simulink model "VDSE_2019b1"  (R2022b)
settings: Solver=ode5  StartTime=0.0  StopTime=T_simulation  FixedStep=simulation_step_time  RelTol=1e-3
values from neighbouring files (symbols this model uses):
  A = 2    [vehicle_parameters_script.m]
  bump_height = 0    [vehicle_parameters_script.m]
  bump_length = 0    [vehicle_parameters_script.m]
  bump_time = 0    [vehicle_parameters_script.m]
  cd = 0.35    [vehicle_parameters_script.m]
  cF = 5000    [vehicle_parameters_script.m]
  clF = -0.15    [vehicle_parameters_script.m]
  clR = -0.20    (= -0.2)    [vehicle_parameters_script.m]
  cp_FA = 30    [vehicle_parameters_script.m]
  cp_RA = 13    [vehicle_parameters_script.m]
  cR = 5000    [vehicle_parameters_script.m]
  ctF = tireF.VERTICAL_DAMPING    [vehicle_parameters_script.m]
  ctR = tireR.VERTICAL_DAMPING    [vehicle_parameters_script.m]
  enableDriverControl = 1    [vehicle_parameters_script.m]
  enableLongDynamics = 1    [vehicle_parameters_script.m]
  enablePowertrain = 1    [vehicle_parameters_script.m]
  g = 9.806    [vehicle_parameters_script.m]
  Gear_numbers = [1 2 3 4 5 6]    [vehicle_parameters_script.m]
  GR = [2.9 1.8 1.3 1 0.85 0.75]    [vehicle_parameters_script.m]
  hcog = 0.441    [vehicle_parameters_script.m]
  hpc = 0.0    (= 0)    [vehicle_parameters_script.m]
  hrcF = 0.3    [vehicle_parameters_script.m]
  hrcg = (hrcF*lR+hrcR*lF)/(lF+lR)    (= 0.25108)    [vehicle_parameters_script.m]
  hrcR = 0.2    [vehicle_parameters_script.m]
  huFcog = 0.32    [vehicle_parameters_script.m]
  huRcog = 0.32    [vehicle_parameters_script.m]
  i1 = 11.42    [vehicle_parameters_script.m]
  i2 = 3.727    [vehicle_parameters_script.m]
  initial_gear = 1    [vehicle_parameters_script.m]
  JwF = 2.45    [vehicle_parameters_script.m]
  JwR = 2.45    [vehicle_parameters_script.m]
  Jx = 4.12    [vehicle_parameters_script.m]
  Jy = 109.16    [vehicle_parameters_script.m]
  Jz = 105.13    [vehicle_parameters_script.m]
  kF = 40000    [vehicle_parameters_script.m]
  kR = 35000    [vehicle_parameters_script.m]
  kRF = 0    [vehicle_parameters_script.m]
  kRR = 0    [vehicle_parameters_script.m]
  ktF = tireF.VERTICAL_STIFFNESS    [vehicle_parameters_script.m]
  ktR = tireR.VERTICAL_STIFFNESS    [vehicle_parameters_script.m]
  lF = 1.223    [vehicle_parameters_script.m]
  lR = l-lF    (= 1.277)    [vehicle_parameters_script.m]
  m = 340    [vehicle_parameters_script.m]
  max_pressure = 1000    [vehicle_parameters_script.m]
  maxrpm = 4000    [vehicle_parameters_script.m]
  mF = 45    [vehicle_parameters_script.m]
  minrpm = 1500    [vehicle_parameters_script.m]
  mR = 50    [vehicle_parameters_script.m]
  output_samping_time = 0.001    [vehicle_parameters_script.m]
  phi0 = 0    [vehicle_parameters_script.m]
  phi_dot0 = 0    [vehicle_parameters_script.m]
  psi0 = 0    [vehicle_parameters_script.m]
  psi_dot0 = 0    [vehicle_parameters_script.m]
  RearRatio = 1    [vehicle_parameters_script.m]
  requested_speed = 120/3.6    (= 33.3333333333)    [vehicle_parameters_script.m]
  rF = tireF.UNLOADED_RADIUS    [vehicle_parameters_script.m]
  rho = 1.2    [vehicle_parameters_script.m]
  rR = tireR.UNLOADED_RADIUS    [vehicle_parameters_script.m]
  steer_ratio = 13.25    [vehicle_parameters_script.m]
  TFL = 0    [vehicle_parameters_script.m]
  TFR = 0    [vehicle_parameters_script.m]
  theta0 = 0    [vehicle_parameters_script.m]
  theta_dot0 = 0    [vehicle_parameters_script.m]
  TRL = 0    [vehicle_parameters_script.m]
  TRR = 0    [vehicle_parameters_script.m]
  Vx0 = 0.01/3.6    (= 0.00277777777778)    [vehicle_parameters_script.m]
  Vy0 = 0    [vehicle_parameters_script.m]
  Vz0 = 0    [vehicle_parameters_script.m]
  wF = 1.578    [vehicle_parameters_script.m]
  wR = 1.544    [vehicle_parameters_script.m]
  x0 = 0    [vehicle_parameters_script.m]
  xcog_overall = (2*mR*xR+2*xF*mF+m*xs)/(m+2*mF+2*mR)    (= 1.25626415094)    [vehicle_parameters_script.m]
  y0 = 0    [vehicle_parameters_script.m]
  z0 = 0    [vehicle_parameters_script.m]
  zFL0 = 0    [vehicle_parameters_script.m]
  zFL_dot0 = 0    [vehicle_parameters_script.m]
  zFR0 = 0    [vehicle_parameters_script.m]
  zFR_dot0 = 0    [vehicle_parameters_script.m]
  zRL0 = 0    [vehicle_parameters_script.m]
  zRL_dot0 = 0    [vehicle_parameters_script.m]
  zRR0 = 0    [vehicle_parameters_script.m]
  zRR_dot0 = 0    [vehicle_parameters_script.m]
undefined symbols (not defined in the file or in its folder): Bxf, Bxr, Byf, Byr, Cxf, Cxr, Cyf, Cyr, DiscIntNeverNeededParam, Dxf, Dxr, Dyf, Dyr, exf, exr, eyf, eyr, FNOMINf, FNOMINr, Ldwf, Ldwr, PCX1f, PCX1r, PCY1f, PCY1r, PDX1f, PDX1r, PDX2f, PDX2r, PDY1f, PDY1r, PDY2f, PDY2r, PDY3f, PDY3r, PEX1f, PEX1r, PEX2f, PEX2r, PEX3f, PEX3r, PEX4f, PEX4r, PEY1f, PEY1r, PEY2f, PEY2r, PEY3f, PEY3r, PEY4f, PEY4r, PHX1f, PHX1r, PHX2f, PHX2r, PHY1f, PHY1r, PHY2f, PHY2r, PHY3f ... (+147)
libraries: simulink x55, mfeval_LIB x4, slpidlib x1
(part 6 of 7)

== matlab function VDSE_2019b1/14-DOF VEHICLE MODEL/SUSPENSION/REAR SUSPENSION/SUSPENSION RR/RR/MATLAB Function ==
  data: mR input; wR input; lR input; cR input; kR input; kRR input; ctR input; ktR input; g input; yRR_road input; yRR_road_dot input; zRR_dot_dot output; z input; Vz input; phi input; phi_dot input; theta input; theta_dot input; zRL input; zRR input; zRR_dot input
function zRR_dot_dot = zRR(mR,wR,lR,cR,kR,kRR,ctR,ktR,g,yRR_road,yRR_road_dot,z,Vz,phi,phi_dot,theta,theta_dot,zRL,zRR,zRR_dot)
% Parameters:
% mR = half rear unsprung mass [kg]
% cR = rear damping damping rate [Ns/m]
% kR = rear spring stiffness [N/m]
% kRR = rear antiroll bar stiffness [N/m]
% wR = rear trackwidth [m]
% g = gravitational acceleration [m/s^2]
%
% Annotations:
% z = sprung mass vertical displacement [m]
% Vz = sprung mass vertical velocity [m/s]
% zij = unsprung vertical displacement [m]
% zij_dot = unsprung vertical velocity [m/s]
% zij_dot_dot = unsprung vertical acceleration [m/s^2]
% theta = pitch angle [rad]
% theta_dot = pitch angular velocity [rad/s]
% phi = roll angle [rad]
% phi_dot  = roll angular velocity [rad/s]
% y_rear_road = rear axle's road input displacement [m]
% y_rear_road_dot = rear axle's road input velocity [m/s]
%
% i: F, R = Front, Rear
% j: R, L = Right, Left

% Summation of forces:
sum = -cR*(Vz-zRR_dot-wR/2*phi_dot+lR*theta_dot) - kR*(z-zRR-wR/2*phi+lR*theta)...
    +kRR/wR*(phi - (zRL-zRR)/wR)+ktR*(zRR-yRR_road)+ ctR*(zRR_dot-yRR_road_dot) + mR*g;
% Calculation of RR unsprung mass vertical acceleration:
zRR_dot_dot = -sum/mR; 

end

== matlab function VDSE_2019b1/14-DOF VEHICLE MODEL/EQUATIONS OF MOTION FOR CHASSIS/Vertical Dynamics/VERTICAL DYNAMICS ==
  data: m input; g input; lF input; Vz_dot output; lR input; wF input; wR input; kF input; kR input; cF input; cR input; phi input; phi_dot input; theta input; theta_dot input; zFL input; zFL_dot input; zFR input; zFR_dot input; zRL input; zRL_dot input; zRR input; zRR_dot input; Vx input; Vy input; fFLz_aero input; fFRz_aero input; fRLz_aero input; fRRz_aero input; z input; z_dot input
function Vz_dot = vertical_dynamics(m,g,lF,lR,wF,wR,kF,kR,cF,cR,phi,phi_dot,...
    theta,theta_dot,zFL,zFL_dot,zFR,zFR_dot,zRL,zRL_dot,zRR,zRR_dot,Vx,Vy,...
    fFLz_aero, fFRz_aero, fRLz_aero, fRRz_aero,z,z_dot)
% Parameters:
% m = sprung mass [kg]
% cF = front damping damping rate [Ns/m]
% cR = rear damping damping rate [Ns/m]
% kF = front spring stiffness [N/m]
% kR = rear spring stiffness [N/m]
% lF = front wheel base [m]
% lR = rear wheel base [m]
% wF = front trackwidth [m]
% wR = rear trackwidth [m]
% g = gravitational acceleration [m/s^2]
%
% Annotations:
% z = sprung mass vertical displacement [m]
% Vz = sprung mass vertical velocity [m/s]
% Vz_dot = sprung mass vertical acceleration [m/s^2]
% zij = unsprung vertical displacement [m]
% zij_dot = unsprung vertical velocity [m/s]
% fijz_aero = downforces applied on the chassis [N]
% theta = pitch angle [rad]
% theta_dot = pitch angular velocity [rad/s]
% phi = roll angle [rad]
% phi_dot  = roll angular velocity [rad/s]
% Vy = vehicle's lateral velocity [m/s]
% Vx = vehicle's longitudinal velocity [m/s]
%
% i: F, R = Front, Rear
% j: R, L = Right, Left

% Summation of forces:
sum=cF*(z_dot-zFL_dot+(wF/2)*phi_dot-lF*theta_dot)...
    +cF*(z_dot-zFR_dot-(wF/2)*phi_dot-lF*theta_dot)...
    +cR*(z_dot-zRL_dot+(wR/2)*phi_dot+lR*theta_dot)...
    +cR*(z_dot-zRR_dot-(wR/2)*phi_dot+lR*theta_dot)...
    +kF*(z-zFL+(wF/2)*phi-lF*theta)...
    +kF*(z-zFR-(wF/2)*phi-lF*theta)...
    +kR*(z-zRL+(wR/2)*phi+lR*theta)...
    +kR*(z-zRR-(wR/2)*phi+lR*theta)...
    +m*g+m*Vx*theta_dot-m*Vy*phi_dot...
    +fFLz_aero+fFRz_aero+fRLz_aero+fRRz_aero;

% Calculation of vertical acceleration of sprung mass (including tangential terms):
Vz_dot=-sum/m;
end

== matlab function VDSE_2019b1/14-DOF VEHICLE MODEL/EQUATIONS OF MOTION FOR CHASSIS/Roll Dynamics/ROLL DYNAMICS ==
  data: Jx input; g input; lF input; phi_dot_dot output; lR input; wF input; wR input; kF input; kR input; kRF input; kRR input; cF input; cR input; z input; z_dot input; theta input; theta_dot input; zFL input; zFL_dot input; zFR input; zFR_dot input; zRL input; zRL_dot input; zRR input; zRR_dot input; ay input; hrcg input; hcog input; m input; fFLz_aero input; fFRz_aero input; fRLz_aero input; fRRz_aero input; phi input; phi_dot input
function phi_dot_dot = roll_dynamics(Jx,g,lF,lR,wF,wR,kF,kR,kRF,kRR,cF,cR,z,z_dot,theta,theta_dot,...
    zFL,zFL_dot,zFR,zFR_dot,zRL,zRL_dot,zRR,zRR_dot,ay,hrcg,hcog,m,...
    fFLz_aero,fFRz_aero,fRLz_aero,fRRz_aero,phi,phi_dot)

% Parameters:
% m = sprung mass [kg]
% Jx = roll moment of inertial [kgm^2]
% cF = front damping damping rate [Ns/m]
% cR = rear damping damping rate [Ns/m]
% kF = front spring stiffness [N/m]
% kR = rear spring stiffness [N/m]
% kRF = front antiroll bar stiffness [N/m]
% kRR = front antiroll bar stiffness [N/m]
% lF = front wheel base [m]
% lR = rear wheel base [m]
% wF = front trackwidth [m]
% wR = rear trackwidth [m]
% hrcg = roll center height at the center of gravity [m]
% hcog = height of center of gravity [m]
% g = gravitational acceleration [m/s^2]
%
% Annotations:
% z = sprung mass vertical displacement [m]
% Vz = sprung mass vertical velocity [m/s]
% Vz_dot = sprung mass vertical acceleration [m/s^2]
% zij = unsprung vertical displacement [m]
% zij_dot = unsprung vertical velocity [m/s]
% fijz_aero = downforces applied on the chassis [N]
% theta = pitch angle [rad]
% theta_dot = pitch angular velocity [rad/s]
% phi = roll angle [rad]
% phi_dot  = roll angular velocity [rad/s]
% ay = vehicle's overall lateral acceleration [m/s^2]
%
% i: F, R = Front, Rear
% j: R, L = Right, Left

% Summation of moments:
sumF=(wF/2)*cF*(z_dot-zFL_dot+(wF/2)*phi_dot-lF*theta_dot)...
    -(wF/2)*cF*(z_dot-zFR_dot-(wF/2)*phi_dot-lF*theta_dot)...
    +(wR/2)*cR*(z_dot-zRL_dot+(wR/2)*phi_dot+lR*theta_dot)...
    -(wR/2)*cR*(z_dot-zRR_dot-(wR/2)*phi_dot+lR*theta_dot)...
    +(wF/2)*kF*(z-zFL+(wF/2)*phi-lF*theta)...
    -(wF/2)*kF*(z-zFR-(wF/2)*phi-lF*theta)...
    +(wR/2)*kR*(z-zRL+(wR/2)*phi+lR*theta)...
    -(wR/2)*kR*(z-zRR-(wR/2)*phi+lR*theta)...
    +kRF*(phi-(zFL-zFR)/wF)...
    +kRR*(phi-(zRL-zRR)/wR)-m*(hcog-hrcg)*ay*cos(phi)-m*g*(hcog-hrcg)*sin(phi)...
    -wF*fFLz_aero+wF*fFRz_aero-wR*fRLz_aero+wR*fRRz_aero;

% Roll angular acceleration calculation:
phi_dot_dot=-sumF/(Jx+m*(hcog-hrcg)^2);
end

== matlab function VDSE_2019b1/14-DOF VEHICLE MODEL/EQUATIONS OF MOTION FOR CHASSIS/Pitch Dynamics/PITCH DYNAMICS ==
  data: Jy input; g input; lF input; theta_dot_dot output; lR input; wF input; wR input; kF input; kR input; cF input; cR input; z input; z_dot input; phi input; phi_dot input; zFL input; zFL_dot input; zFR input; zFR_dot input; zRL input; zRL_dot input; zRR input; zRR_dot input; ax input; hpc input; hcog input; m input; fFLz_aero input; fFRz_aero input; fRLz_aero input; fRRz_aero input; theta input; theta_dot input
function theta_dot_dot = pitch_dynamics(Jy,g,lF,lR,wF,wR,kF,kR,cF,cR,z,z_dot,phi,phi_dot,...
    zFL,zFL_dot,zFR,zFR_dot,zRL,zRL_dot,zRR,zRR_dot,ax,hpc,hcog,m,...
    fFLz_aero,fFRz_aero,fRLz_aero,fRRz_aero,theta, theta_dot)
% Parameters:
% m = sprung mass [kg]
% Jy = pitch moment of inertial [kgm^2]
% cF = front damping damping rate [Ns/m]
% cR = rear damping damping rate [Ns/m]
% kF = front spring stiffness [N/m]
% kR = rear spring stiffness [N/m]
% lF = front wheel base [m]
% lR = rear wheel base [m]
% wF = front trackwidth [m]
% wR = rear trackwidth [m]
% hpc = pitch center height at the center of gravity [m]
% hcog = height of center of gravity [m]
% g = gravitational acceleration [m/s^2]
%
% Annotations:
% z = sprung mass vertical displacement [m]
% Vz = sprung mass vertical velocity [m/s]
% Vz_dot = sprung mass vertical acceleration [m/s^2]
% zij = unsprung vertical displacement [m]
% zij_dot = unsprung vertical velocity [m/s]
% fijz_aero = downforces applied on the chassis [N]
% theta = pitch angle [rad]
% theta_dot = pitch angular velocity [rad/s]
% phi = roll angle [rad]
% phi_dot  = roll angular velocity [rad/s]
% ax = vehicle's overall longitudinal acceleration [m/s^2]
%
% i: F, R = Front, Rear
% j: R, L = Right, Left

% Summation of moments:
sumF=-lF*cF*(z_dot-zFL_dot+(wF/2)*phi_dot-lF*theta_dot)...
    -lF*cF*(z_dot-zFR_dot-(wF/2)*phi_dot-lF*theta_dot)...
    +lR*cR*(z_dot-zRL_dot+(wR/2)*phi_dot+lR*theta_dot)...
    +lR*cR*(z_dot-zRR_dot-(wR/2)*phi_dot+lR*theta_dot)...
    -lF*kF*(z-zFL+(wF/2)*phi-lF*theta)...
    -lF*kF*(z-zFR-(wF/2)*phi-lF*theta)...
    +lR*kR*(z-zRL+(wR/2)*phi+lR*theta)...
    +lR*kR*(z-zRR-(wR/2)*phi+lR*theta)-m*(hcog-hpc)*ax*cos(theta)-m*g*(hcog-hpc)*sin(theta)...
    -lF*fFLz_aero-lF*fFRz_aero+lR*fRLz_aero+lR*fRRz_aero;
      
theta_dot_dot=-sumF/(Jy+m*(hcog-hpc)^2);
end

== matlab function VDSE_2019b1/14-DOF VEHICLE MODEL/WHEEL ASSEMBLY/WHEEL ASSEMBLY BCD/TIRE FORCES AND WHEEL DYNAMICS ==
  data: rF input; rR input; JwF input; JwR input; fFLz input; fFRz input; fRLz input; fRRz input; omegaFL input; omegaFR input; omegaRL input; omegaRR input; fFLx output; fFRx output; fRLx output; fRRx output; VFLx input; VFLy input; VFRx input; VFRy input; VRLx input; VRLy input; VRRx input; VRRy input; fFLy output; fFRy output; fRLy output; fRRy output; omega_dot output size=[1 4]; TFL input; TFR input; TRL input; TRR input; TireParams input
function [fFLx, fFRx, fRLx,fRRx, fFLy,  fFRy, fRLy, fRRy, omega_dot] = TIRES(rF, rR, JwF, JwR,...
    fFLz, fFRz, fRLz, fRRz,...
    omegaFL, omegaFR, omegaRL, omegaRR, ...
    VFLx, VFLy, VFRx, VFRy, VRLx, VRLy, VRRx, VRRy, TFL, TFR, TRL, TRR, TireParams)
% Longitudinal slip:
sFLx = (VFLx - omegaFL*rF)/abs(omegaFL*rF);
sFRx = (VFRx - omegaFR*rF)/abs(omegaFR*rF);
sRLx = (VRLx - omegaRL*rR)/abs(omegaRL*rR);
sRRx = (VRRx - omegaRR*rR)/abs(omegaRR*rR);


% Lateral slip:
if VFLx==0
    sFLy = 0;
else
    sFLy = (1 + sFLx)*VFLy/abs(VFLx);
end

if VFRx==0
    sFRy = 0;
else
    sFRy = (1 + sFRx)*VFRy/abs(VFRx);
end

if VRLx==0
    sRLy = 0;
else
    sRLy = (1 + sRLx)*VRLy/abs(VRLx);
end

if VRRx == 0
    sRRy = 0;
else
 
    sRRy = (1 + sRRx)*VRRy/abs(VRRx);
end

% Total slip:
sFL = sqrt(sFLx^2 + sFLy^2);
sFR = sqrt(sFRx^2 + sFRy^2);
sRL = sqrt(sRLx^2 + sRLy^2);
sRR = sqrt(sRRx^2 + sRRy^2);

%Tire parameters
Bxf = TireParams(1);
Cxf = TireParams(2);
Dxf = TireParams(3);
Bxr = TireParams(4);
Cxr = TireParams(5);
Dxr = TireParams(6);
Byf = TireParams(7);
Cyf = TireParams(8);
Dyf = TireParams(9);
Byr = TireParams(10);
Cyr = TireParams(11);
Dyr = TireParams(12);

% BCD Version - Longitudinal:
muFLx = Dxf*sin(Cxf*atan(Bxf*sFL));
muFRx = Dxf*sin(Cxf*atan(Bxf*sFR));
muRLx = Dxr*sin(Cxr*atan(Bxr*sRL));
muRRx = Dxr*sin(Cxr*atan(Bxr*sRR));


% % BCD Version - Lateral:
muFLy = Dyf*sin(Cyf*atan(Byf*sFL));
muFRy = Dyf*sin(Cyf*atan(Byf*sFR));
muRLy = Dyr*sin(Cyr*atan(Byr*sRL));
muRRy = Dyr*sin(Cyr*atan(Byr*sRR));


if sFL == 0
muFLx_long = 0;
muFLy_lat = 0;
else
muFLx_long = -sFLx*muFLx/sFL;
muFLy_lat = -sFLy*muFLy/sFL;
end

if sFR == 0
muFRx_long = 0;
muFRy_lat = 0;
else
muFRx_long = -sFRx*muFRx/sFR;
muFRy_lat = -sFRy*muFRy/sFR;
end

if sRL == 0
muRLx_long = 0;
muRLy_lat = 0;
else
muRLx_long = -sRLx*muRLx/sRL;
muRLy_lat = -sRLy*muRLy/sRL;
end

if sRR == 0
muRRx_long = 0;
muRRy_lat = 0;
else    
muRRx_long = -sRRx*muRRx/sRR;
muRRy_lat = -sRRy*muRRy/sRR;
end

fFLx = fFLz*muFLx_long; fFLy = fFLz*muFLy_lat;
fFRx = fFRz*muFRx_long; fFRy = fFRz*muFRy_lat;
fRLx = fRLz*muRLx_long; fRLy = fRLz*muRLy_lat;
fRRx = fRRz*muRRx_long; fRRy = fRRz*muRRy_lat;

%Wheel Dynamics
domegaFL = (TFL - fFLx*rF)/(JwF);
domegaFR = (TFR - fFRx*rF)/(JwF);
domegaRL = (TRL - fRLx*rR)/(JwR);
domegaRR = (TRR - fRRx*rR)/(JwR);

omega_dot = [domegaFL, domegaFR, domegaRL, domegaRR];

end

== matlab function VDSE_2019b1/14-DOF VEHICLE MODEL/WHEEL ASSEMBLY/WHEEL ASSEMBLY BCD/TIRE VELOCITIES ==
  data: deltaFL input; VFLx output; VFLy output; VFRx output; VFRy output; VRLx output; VRLy output; VRRx output; deltaFR input; deltaRL input; deltaRR input; V input; beta input; psidot input; lF input; lR input; VRRy output; wFL input; wFR input; wRL input; wRR input
function [VFLx, VFLy, VFRx, VFRy, VRLx, VRLy, VRRx, VRRy] = ConversiontoCorners(deltaFL,deltaFR,deltaRL,deltaRR,...
    V, beta, psidot,  lF, lR, wFL, wFR, wRL, wRR)
% Geometric calcs
lFL = sqrt(lF^2+wFL^2); gammaFL = atan2(wFL,lF);
lFR = sqrt(lF^2+wFR^2); gammaFR = atan2(wFR,lF);
lRL = sqrt(lR^2+wRL^2); gammaRL = atan2(wRL,lR);
lRR = sqrt(lR^2+wRR^2); gammaRR = atan2(wRR,lR);

% Tire Velocities
VFLx = V*cos(deltaFL - beta) - psidot*lFL*sin(gammaFL - deltaFL);
VFLy = - V*sin(deltaFL - beta) + psidot*lFL*cos(gammaFL - deltaFL);
VFRx = V*cos(deltaFR - beta) + psidot*lFR*sin(gammaFR + deltaFR);
VFRy = - V*sin(deltaFR - beta) + psidot*lFR*cos(gammaFR + deltaFR);
VRLx = V*cos(deltaRL - beta) - psidot*lRL*sin(gammaRL + deltaRL);
VRLy = -V*sin(deltaRL - beta) - psidot*lRL*cos(gammaRL + deltaRL);
VRRx = V*cos(deltaRR - beta) + psidot*lRR*sin(gammaRR - deltaRR);
VRRy = -V*sin(deltaRR - beta) - psidot*lRR*cos(gammaRR - deltaRR);
end

== matlab function VDSE_2019b1/14-DOF VEHICLE MODEL/EQUATIONS OF MOTION FOR CHASSIS/Longitudinal Dynamics/LONGIDUTINAL DYNAMICS ==
  data: deltaFL input; ax output; fFLx input; fFLy input; deltaFR input; fFRx input; fFRy input; deltaRL input; fRLx input; fRLy input; deltaRR input; fRRx input; fRRy input; mFLy input; mFRy input; mRLy input; mRRy input; Vy input; psi_dot input; theta_dot input; Vz input; Vx input; m input; mF input; mR input; rho input; cd input; A input; rF input; rR input; Vx_dot output
function [ax, Vx_dot] = longitudinal_dynamics(deltaFL, fFLx, fFLy, deltaFR, fFRx, fFRy, deltaRL, fRLx, fRLy, deltaRR, fRRx, fRRy,mFLy,mFRy,mRLy,mRRy, ...
    Vy, psi_dot, theta_dot, Vz, Vx, m, mF, mR,rho,cd,A,rF,rR)

% Parameters:
% m = sprung mass [kg]
% mF = half front unsprung mass [kg]
% mR = half rear unsprung mass [kg]
% rho = air density [kg/m^3]
% cd = drag coefficient [-]
% A = vehicle's frontal area [m^2]
% rF = front dynamic radius [m]
% rR = rear dynamic radius [m]
%
% Annotations:
% fijx, fijy = force at the tire frame [N]
% mijy = rolling moment at the tire frame [Nm]
% ax = overall longidutinal acceleration [m/s^2]
% Vx_dot = longidutinal acceleration excluding tangential terms [m/s^2]
% theta_dot = pitch angular velocity [rad/s]
% psi_dot = yaw angular velocity [rad/s]
% Vz = vertical sprung mass velocity [m/s]
% Vy = lateral vehicle's velocity [m/s]
% Vx = longitudinal vehicle's velocity [m/s]
% deltaFL = FL wheel's steering angle [rad]
% deltaFR = FR wheel's steering angle [rad]
% deltaRL = RL wheel's steering angle [rad]
% deltaRR = RR wheel's steering angle [rad]
%
% i: F, R = Front, Rear
% j: R, L = Right, Left

% Projection in the vehicle frame:
fFLx_vehicle=fFLx*cos(deltaFL)-fFLy*sin(deltaFL);  
fFRx_vehicle=fFRx*cos(deltaFR)-fFRy*sin(deltaFR);
fRLx_vehicle=fRLx*cos(deltaRL)-fRLy*sin(deltaRL);
fRRx_vehicle=fRRx*cos(deltaRR)-fRRy*sin(deltaRR);

% Calculation of overall longitudinal acceleration:
ax = (fFLx_vehicle+fFRx_vehicle+fRLx_vehicle+fRRx_vehicle+mFLy/rF*cos(deltaFL)+mFRy/rF*cos(deltaFR)+...
    mRLy/rR*cos(deltaRL)+mRRy/rR*cos(deltaRR)-1/2*rho*cd*A*Vx^2)/(m+2*mR+2*mF);

% Calculation of vehicle's longitudinal acceleration excluding tangential terms: 
Vx_dot = ax - theta_dot*Vz + Vy*psi_dot;

end

== matlab function VDSE_2019b1/14-DOF VEHICLE MODEL/WHEEL ASSEMBLY/WHEEL ASSEMBLY PACEIJKA/TIRE FORCES AND WHEEL DYNAMICS ==
  data: rF input; rR input; JwF input; JwR input; fFLz input; fFRz input; fRLz input; fRRz input; omegaFL input; omegaFR input; omegaRL input; omegaRR input; fFLx output; fFRx output; fRLx output; fRRx output; VFLx input; VFLy input; VFRx input; VFRy input; VRLx input; VRLy input; VRRx input; VRRy input; fFLy output; fFRy output; fRLy output; fRRy output; mFLz output; mFRz output; mRLz output; mRRz output; mFLy output; mFRy output; mRLy output; mRRy output; omega_dot output size=[1 4]; TFL input; TFR input; TRL input; TRR input; gammaFL input; gammaFR input; gammaRL input; gammaRR input; TireParams_front input; TireParams_rear input
function [fFLx, fFRx, fRLx,fRRx, fFLy,  fFRy, fRLy, fRRy, mFLz, mFRz, mRLz, mRRz,...
    mFLy, mFRy, mRLy, mRRy, omega_dot] = TIRES(rF, rR, JwF, JwR,...
    fFLz, fFRz, fRLz, fRRz,...
    omegaFL, omegaFR, omegaRL, omegaRR, ...
    VFLx, VFLy, VFRx, VFRy, VRLx, VRLy, VRRx, VRRy, TFL, TFR, TRL, TRR,...
    gammaFL, gammaFR, gammaRL, gammaRR, ...
    TireParams_front, TireParams_rear)
FzFL = fFLz; FzFR = fFRz;FzRL = fRLz;FzRR = fRRz;
%% Longitudinal Slip Calculation
sFLx = -(VFLx - omegaFL*rF)/VFLx;
sFRx = -(VFRx - omegaFR*rF)/VFRx;
sRLx = -(VRLx - omegaRL*rR)/VRLx;
sRRx = -(VRRx - omegaRR*rR)/VRRx;
%% Lateral slip Calculation
if VFLx==0
    sFLy = 0;
else
    sFLy = atan(VFLy/abs(VFLx));
end

if VFRx==0
    sFRy = 0;
else
    sFRy = atan(VFRy/abs(VFRx));
end

if VRLx==0
    sRLy = 0;
else
    sRLy = atan(VRLy/abs(VRLx));
end

if VRRx == 0
    sRRy = 0;
else

    sRRy = atan(VRRy/abs(VRRx));
end

%% Tire Parameters for Front Axle
pHx1 = TireParams_front(1);
pHx2 = TireParams_front(2);
pDx1 = TireParams_front(3);
pDx2 = TireParams_front(4);
pCx1 = TireParams_front(5);
pEx1 = TireParams_front(6);
pEx2 = TireParams_front(7);
pEx3 = TireParams_front(8);
pEx4 = TireParams_front(9);
pKx1 = TireParams_front(10);
pKx2 = TireParams_front(11);
pKx3 = TireParams_front(12);
ex   =  TireParams_front(13);
pVx1 = TireParams_front(14);
pVx2 = TireParams_front(15);
pKy1 = TireParams_front(16);
pKy2 = TireParams_front(17);
pKy3 = TireParams_front(18);
pVy1 = TireParams_front(19);
pVy2 = TireParams_front(20);
pVy3 = TireParams_front(21);
pVy4 = TireParams_front(22);
pHy1 = TireParams_front(23);
pHy2 = TireParams_front(24);
pHy3 = TireParams_front(25);
pDy1 = TireParams_front(26);
pDy2 = TireParams_front(27);
pDy3 = TireParams_front(28);
pCy1 = TireParams_front(29);
pEy1 = TireParams_front(30);
pEy2 = TireParams_front(31);
pEy3 = TireParams_front(32);
pEy4 = TireParams_front(33);
ey = TireParams_front(34);
rBx1 = TireParams_front(35);
rBx2 = TireParams_front(36);
rCx1 = TireParams_front(37);
rEx1 = TireParams_front(38);
rEx2 = TireParams_front(39);
rHx1 = TireParams_front(40);
rBy1 = TireParams_front(41);
rBy2 = TireParams_front(42);
rBy3 = TireParams_front(43);
rCy1 = TireParams_front(44);
rVy1 = TireParams_front(45);
rVy2 = TireParams_front(46);
rVy3 = TireParams_front(47);
rVy4 = TireParams_front(48);
rVy5 = TireParams_front(49);
rVy6 = TireParams_front(50);
rEy1 = TireParams_front(51);
rEy2 = TireParams_front(52);
rHy1 = TireParams_front(53);
rHy2 = TireParams_front(54);
FzFL0 = TireParams_front(55);
FzFR0 = TireParams_front(55);
qHz1 = TireParams_front(56);
qHz2 = TireParams_front(57);
qHz3 = TireParams_front(58);
qHz4 = TireParams_front(59);
qBz1 = TireParams_front(60);
qBz2 = TireParams_front(61);
qBz3 = TireParams_front(62);
qBz4 = TireParams_front(63);
qBz5 = TireParams_front(64);
qCz1 = TireParams_front(65);
qDz1 = TireParams_front(66);
qDz2 = TireParams_front(67);
qDz3 = TireParams_front(68);
qDz4 = TireParams_front(69);
qEz1 = TireParams_front(70);
qEz2 = TireParams_front(71);
qEz3 = TireParams_front(72);
qEz4 = TireParams_front(73);
qEz5 = TireParams_front(74);
qBz9 = TireParams_front(75);
qBz10 = TireParams_front(76);
qDz6 = TireParams_front(77);
qDz7 = TireParams_front(78);
qDz8 = TireParams_front(79);
qDz9 = TireParams_front(80);
R0 = TireParams_front(81);
z7 = TireParams_front(82);
ssz1 = TireParams_front(83);
ssz2 = TireParams_front(84);
ssz3 = TireParams_front(85);
ssz4 = TireParams_front(86);
qsy1 = TireParams_front(87);
qsy2 = TireParams_front(88);
qsy3 = TireParams_front(89);
qsy4 = TireParams_front(90);
Vref = TireParams_front(91);
epsilonk = 10e-12;
%% Deviation
dFzFL = (FzFL - FzFL0)/FzFL0;
dFzFR = (FzFR - FzFR0)/FzFR0;
%% Front Left Tire
%-------------------------------------------------------------------------%
%                      PURE LONGITUDINAL                    %
%-------------------------------------------------------------------------%
% Horizontal offset to the force/slip function of load
ShxFL   = pHx1 + pHx2.*dFzFL; 
% kxFL     = sFLx;
% Longitudinal coefficient of friction in function of load
mux1FL  = (pDx1 + pDx2.*dFzFL); 
% Peak factor
DxFL    = mux1FL*FzFL; 
% Longitudinal slip ratio with offset
KxFL    = sFLx + ShxFL; 
% Shape factor
CxFL    = pCx1; 
% Curvature factor function of load
ExFL    = (pEx1 + pEx2*dFzFL + pEx3*dFzFL*dFzFL)*(1 - pEx4*sign(KxFL)); 
% Slip stiffness Kfx/Fz function of load
KxkFL   = FzFL*(pKx1 + pKx2.*dFzFL)*exp(pKx3.*dFzFL); 
% Stiffness factor
BxFL    = KxkFL/(CxFL*DxFL + ex); 
% Vertical offset to the force/slip function of load
SVxFL   = FzFL.*(pVx1 + pVx2.*dFzFL); 
% Longitudinal Force:
Fx0FL = DxFL*sin(CxFL*atan(BxFL*KxFL - ExFL*(BxFL*KxFL - atan(BxFL*KxFL)))) + SVxFL;

%-------------------------------------------------------------------------%
%                      PURE LATERAL                    %
%-------------------------------------------------------------------------%
% Slip stiffness Kfx/Fz function of load
% Kyalf   = pKy1.*Fztlf0.*sin(pKy4.*atan(Fztlf./(pKy2+pKy5.*gammalf.^2)./Fztlf0))./(1+pKy3.*abs(gammalf));  % from book 
KyaFL = pKy1*FzFL0*sin(2*atan(FzFL/(pKy2*FzFL0)))*(1-pKy3*abs(gammaFL)); %Instead of sign, I put abs
% Kyglf   = (pKy6 + pKy7.*dFztlf).*Fztlf;
% Vertical offset to the force/slip function of load
SVygFL  = FzFL.*(pVy3 + pVy4.*dFzFL)*gammaFL;
SVyFL   = FzFL.*(pVy1 + pVy2.*dFzFL) + SVygFL; 
% Horizontal offset to the force/slip function of load
% Shlfy   = (pHy1 + pHy2.*dFztlf)+ (Kyglf.*gammalf - Svyglf)./(Kyalf +10^-6); %from book
SHyFL = (pHy1 + pHy2*dFzFL) + pHy3.*gammaFL; %from Carmaker
% Lateral coefficient of friction in function of load
muy1FL  = (pDy1 + pDy2*dFzFL)/(1 - pDy3*gammaFL^2);
% Peak factor
DyFL    = muy1FL*FzFL; 
% Lateral slip ratio
ayFL    = sFLy + SHyFL; 
% Shape factor
CyFL    = pCy1; 
% Curvature factor function of load
EyFL    = (pEy1 + pEy2*dFzFL)*(1 - (pEy3+pEy4*gammaFL)*sign(ayFL)); 
% Stiffness factor
ByFL    = KyaFL/(CyFL*DyFL + ey); 
% Lateral Force:
Fy0FL = DyFL*sin(CyFL*atan(ByFL*ayFL - EyFL*(ByFL*ayFL - atan(ByFL*ayFL)))) + SVyFL;

%-------------------------------------------------------------------------%
%                    COMBINED LONGITUDINAL                  %
%-------------------------------------------------------------------------%
BxaFL = rBx1*cos(atan(rBx2*sFLx));
CxaFL = rCx1;
ExaFL = rEx1 + rEx2*dFzFL;
SHxaFL = rHx1;
aFL = sFLy + SHxaFL;
Gxa0FL = cos(CxaFL*(atan(BxaFL*SHxaFL - ExaFL*(BxaFL*SHxaFL - atan(BxaFL*SHxaFL)))));
GxaFL = (cos(CxaFL*(atan(BxaFL*aFL - ExaFL*(BxaFL*aFL - atan(BxaFL*aFL))))))/Gxa0FL;
fFLx = GxaFL*Fx0FL;

%-------------------------------------------------------------------------%
%                       COMBINED LATERAL                     %
%-------------------------------------------------------------------------%

BykFL = rBy1*cos(atan(rBy2*(sFLy-rBy3)));
CykFL = rCy1;
DVykFL = muy1FL*FzFL*(rVy1+rVy2*dFzFL + rVy3*gammaFL)*cos(atan(rVy4*sFLy));
EykFL = rEy1 + rEy2*dFzFL;
SHykFL = rHy1 + rHy2*dFzFL;
SVykFL = DVykFL.*sin(rVy5*atan(rVy6*sFLx));
KsFL = sFLx + SHykFL;
Gy0kFL = cos(CykFL*atan(BykFL*SHykFL - EykFL*(BykFL*SHykFL - atan(BykFL*SHykFL))));
GykFL = cos(CykFL*atan(BykFL*KsFL - EykFL*(BykFL*KsFL - atan(BykFL*KsFL))))/Gy0kFL;
fFLy = GykFL*Fy0FL+SVykFL;


%-------------------------------------------------------------------------%
%                       PURE ALIGNING TORQUE                     %
%-------------------------------------------------------------------------%

Dr = FzFL*R0*((qDz6+qDz7*dFzFL)+(qDz8+qDz9*dFzFL)*gammaFL)-1;
SHtFL = qHz1+ qHz2*dFzFL+(qHz3+qHz4*dFzFL)*gammaFL;
at = sFLy + SHtFL;
Br = (qBz9+qBz10*ByFL*CyFL);
Dt0 = FzFL*(R0/FzFL0)*(qDz1+qDz2*dFzFL);
Dt = Dt0*(1+qDz3*gammaFL+qDz4*gammaFL^2);
Ct = qCz1;
Bt = (qBz1+qBz2*dFzFL+qBz3*dFzFL^2)*(1+qBz4*gammaFL+qBz5*abs(gammaFL));
Et = (qEz1+qEz2*dFzFL+qEz3*dFzFL^2)*(1+(qEz4+qEz5*gammaFL)*2/pi*atan(Bt*Ct*at));
Kya_primeFL = KyaFL+epsilonk;
SHfFL = SHyFL + SVyFL/Kya_primeFL;
ar = sFLy+SHfFL;
Cr = z7;
Mzr0FL = Dr*cos(Cr*atan(Br*ar))*cos(sFLy);
t0FL = Dt*cos(Ct*atan(Bt*at - Et*(Bt*at - atan(Bt*at))))*cos(sFLy);
Mz0_primeFL = -t0FL*Fy0FL;
Mz0FL = Mz0_primeFL + Mzr0FL;


%-------------------------------------------------------------------------%
%                       COMBINED ALIGNING TORQUE             %
%-------------------------------------------------------------------------%

areg = atan(sqrt(tan(ar)^2+(KxkFL/Kya_primeFL)^2*sFLx^2))*sign(ar);
ateg = atan(sqrt(tan(at)^2+(KxkFL/Kya_primeFL)^2*sFLx^2))*sign(at);
s = R0*(ssz1+ssz2*(fFLy/FzFL0)+(ssz3+ssz4*dFzFL))*gammaFL;
MzrFL = Dr*cos(Cr*atan(Br*areg))*cos(sFLy);
Fy_primeFL = fFLy - SVykFL;
t = Dt*cos(Ct*atan(Bt*ateg-Et*(Bt*ateg - atan(Bt*ateg))))*cos(sFLy);
Mz_primeFL = -t*Fy_primeFL;
mFLz = Mz_primeFL+MzrFL+s*fFLx;

%-------------------------------------------------------------------------%
%                       ROLLING RESISTANCE TORQUE             %
%-------------------------------------------------------------------------%

mFLy = -FzFL*R0*(qsy1+qsy2*(fFLx/FzFL0)+qsy3*(VFLx/Vref)+qsy4*(VFLx/Vref)^4);

%% Front Right Tire

%-------------------------------------------------------------------------%
%                      PURE LONGITUDINAL                    %
%-------------------------------------------------------------------------%
% Horizontal offset to the force/slip function of load
ShxFR   = pHx1 + pHx2.*dFzFR; 
% Longitudinal coefficient of friction in function of load
mux1FR  = (pDx1 + pDx2.*dFzFR); 
% Peak factor
DxFR    = mux1FR*FzFR; 
% Longitudinal slip ratio with offset
KxFR    = sFRx + ShxFR; 
% Shape factor
CxFR   = pCx1; 
% Curvature factor function of load
ExFR    = (pEx1 + pEx2*dFzFR + pEx3*dFzFR*dFzFR)*(1 - pEx4.*sign(KxFR)); 
% Slip stiffness Kfx/Fz function of load
KxkFR   = FzFR*(pKx1 + pKx2.*dFzFR)*exp(pKx3.*dFzFR); 
% Stiffness factor
BxFR    = KxkFR/(CxFR*DxFR + ex); 
% Vertical offset to the force/slip function of load
SVxFR   = FzFR.*(pVx1 + pVx2.*dFzFR); 
% Longitudinal Force:
Fx0FR = DxFR*sin(CxFR*atan(BxFR*KxFR - ExFR*(BxFR*KxFR - atan(BxFR*KxFR)))) + SVxFR;

%-------------------------------------------------------------------------%
%                      PURE LATERAL                    %
%-------------------------------------------------------------------------%
% Slip stiffness Kfx/Fz function of load
% Kyalf   = pKy1.*Fztlf0.*sin(pKy4.*atan(Fztlf./(pKy2+pKy5.*gammalf.^2)./Fztlf0))./(1+pKy3.*abs(gammalf));  % from book 
KyaFR = pKy1.*FzFR0.*sin(2*atan(FzFR/(pKy2*FzFR0)))*(1-pKy3*abs(gammaFR)); %Instead of sign, I put abs
% Kyglf   = (pKy6 + pKy7.*dFztlf).*Fztlf;
% Vertical offset to the force/slip function of load
SVygFR  = FzFR.*(pVy3 + pVy4.*dFzFR).*gammaFR;
SVyFR   = FzFR.*(pVy1 + pVy2.*dFzFR) + SVygFR; 
% Horizontal offset to the force/slip function of load
% Shlfy   = (pHy1 + pHy2.*dFztlf)+ (Kyglf.*gammalf - Svyglf)./(Kyalf +10^-6); %from book
SHyFR = (pHy1 + pHy2.*dFzFR) + pHy3.*gammaFR; %from Carmaker
% Lateral coefficient of friction in function of load
muy1FR  = (pDy1 + pDy2*dFzFR)/(1 - pDy3.*gammaFR^2);
% Peak factor
DyFR    = muy1FR*FzFR; 
% Lateral slip ratio
ayFR    = sFRy + SHyFR; 
% Shape factor
CyFR    = pCy1; 
% Curvature factor function of load
EyFR    = (pEy1 + pEy2.*dFzFR).*(1 -(pEy3+pEy4.*gammaFR).*sign(ayFR)); 
% Stiffness factor
ByFR    = KyaFR/(CyFR*DyFR + ey); 
% Lateral Force:
Fy0FR = DyFR*sin(CyFR*atan(ByFR*ayFR - EyFR*(ByFR*ayFR - atan(ByFR*ayFR)))) + SVyFR;

%-------------------------------------------------------------------------%
%                    COMBINED LONGITUDINAL                  %
%-------------------------------------------------------------------------%
BxaFR = rBx1.*cos(atan(rBx2.*sFRx));
CxaFR = rCx1;
ExaFR = rEx1 + rEx2.*dFzFR;
SHxaFR = rHx1;
aFR = sFRy + SHxaFR;
Gxa0FR = cos(CxaFR*(atan(BxaFR*SHxaFR - ExaFR*(BxaFR*SHxaFR - atan(BxaFR*SHxaFR)))));
GxaFR = (cos(CxaFR*(atan(BxaFR*aFR - ExaFR*(BxaFR*aFR - atan(BxaFR*aFR))))))/Gxa0FR;
fFRx = GxaFR*Fx0FR;

%-------------------------------------------------------------------------%
%                       COMBINED LATERAL                     %
%-------------------------------------------------------------------------%

BykFR = rBy1*cos(atan(rBy2*(sFRy-rBy3)));
CykFR = rCy1;
DVykFR = muy1FR*FzFR*(rVy1+rVy2*dFzFR + rVy3*gammaFR)*cos(atan(rVy4*sFRy));
EykFR = rEy1 + rEy2*dFzFR;
SHykFR = rHy1 + rHy2*dFzFR;
SVykFR= DVykFR*sin(rVy5*atan(rVy6*sFRx));
KsFR = sFRx + SHykFR;
Gy0kFR = cos(CykFR*atan(BykFR*SHykFR - EykFR*(BykFR*SHykFR - atan(BykFR*SHykFR))));
GykFR = cos(CykFR*atan(BykFR*KsFR - EykFR*(BykFR*KsFR - atan(BykFR*KsFR))))/Gy0kFR;
fFRy = GykFR*Fy0FR+SVykFR;


%-------------------------------------------------------------------------%
%                       PURE ALIGNING TORQUE                     %
%-------------------------------------------------------------------------%

Dr = FzFR*R0*((qDz6+qDz7*dFzFR)+(qDz8+qDz9*dFzFR)*gammaFR)-1;
SHtFR = qHz1+ qHz2*dFzFR+(qHz3+qHz4*dFzFR)*gammaFR;
at = sFRy + SHtFR;
Br = (qBz9+qBz10*ByFR*CyFR);
Dt0 = FzFR*(R0/FzFR0)*(qDz1+qDz2*dFzFR);
Dt = Dt0*(1+qDz3*gammaFR+qDz4*gammaFR^2);
Ct = qCz1;
Bt = (qBz1+qBz2*dFzFR+qBz3*dFzFR^2)*(1+qBz4*gammaFR+qBz5*abs(gammaFR));
Et = (qEz1+qEz2*dFzFR+qEz3*dFzFR^2)*(1+(qEz4+qEz5*gammaFR)*2/pi*atan(Bt*Ct*at));
Kya_primeFR = KyaFR+epsilonk;
SHfFR = SHyFR + SVyFR/Kya_primeFR;
ar = sFRy+SHfFR;
Cr = z7;
Mzr0FR = Dr*cos(Cr*atan(Br*ar))*cos(sFRy);
t0FR = Dt*cos(Ct*atan(Bt*at - Et*(Bt*at - atan(Bt*at))))*cos(sFRy);
Mz0_primeFR = -t0FR*Fy0FR;
Mz0FR = Mz0_primeFR + Mzr0FR;


%-------------------------------------------------------------------------%
%                       COMBINED ALIGNING TORQUE             %
%-------------------------------------------------------------------------%

areg = atan(sqrt(tan(ar)^2+(KxkFR/Kya_primeFR)^2*sFRx^2))*sign(ar);
ateg = atan(sqrt(tan(at)^2+(KxkFR/Kya_primeFR)^2*sFRx^2))*sign(at);
s = R0*(ssz1+ssz2*(fFRy/FzFR0)+(ssz3+ssz4*dFzFR))*gammaFR;
MzrFR = Dr*cos(Cr*atan(Br*areg))*cos(sFRy);
Fy_primeFR = fFRy - SVykFR;
t = Dt*cos(Ct*atan(Bt*ateg-Et*(Bt*ateg - atan(Bt*ateg))))*cos(sFRy);
Mz_primeFR = -t*Fy_primeFR;
mFRz = Mz_primeFR+MzrFR+s*fFRx;

%-------------------------------------------------------------------------%
%                       ROLLING RESISTANCE TORQUE             %
%-------------------------------------------------------------------------%

mFRy = -FzFR*R0*(qsy1+qsy2*(fFRx/FzFR0)+qsy3*(VFRx/Vref)+qsy4*(VFRx/Vref)^4);


%% Tire Parameters for Rear Axle
pHx1 = TireParams_rear(1);
pHx2 = TireParams_rear(2);
pDx1 = TireParams_rear(3);
pDx2 = TireParams_rear(4);
pCx1 = TireParams_rear(5);
pEx1 = TireParams_rear(6);
pEx2 = TireParams_rear(7);
pEx3 = TireParams_rear(8);
pEx4 = TireParams_rear(9);
pKx1 = TireParams_rear(10);
pKx2 = TireParams_rear(11);
pKx3 = TireParams_rear(12);
ex   =  TireParams_rear(13);
pVx1 = TireParams_rear(14);
pVx2 = TireParams_rear(15);
pKy1 = TireParams_rear(16);
pKy2 = TireParams_rear(17);
pKy3 = TireParams_rear(18);
pVy1 = TireParams_rear(19);
pVy2 = TireParams_rear(20);
pVy3 = TireParams_rear(21);
pVy4 = TireParams_rear(22);
pHy1 = TireParams_rear(23);
pHy2 = TireParams_rear(24);
pHy3 = TireParams_rear(25);
pDy1 = TireParams_rear(26);
pDy2 = TireParams_rear(27);
pDy3 = TireParams_rear(28);
pCy1 = TireParams_rear(29);
pEy1 = TireParams_rear(30);
pEy2 = TireParams_rear(31);
pEy3 = TireParams_rear(32);
pEy4 = TireParams_rear(33);
ey = TireParams_rear(34);
rBx1 = TireParams_rear(35);
rBx2 = TireParams_rear(36);
rCx1 = TireParams_rear(37);
rEx1 = TireParams_rear(38);
rEx2 = TireParams_rear(39);
rHx1 = TireParams_rear(40);
rBy1 = TireParams_rear(41);
rBy2 = TireParams_rear(42);
rBy3 = TireParams_rear(43);
rCy1 = TireParams_rear(44);
rVy1 = TireParams_rear(45);
rVy2 = TireParams_rear(46);
rVy3 = TireParams_rear(47);
rVy4 = TireParams_rear(48);
rVy5 = TireParams_rear(49);
rVy6 = TireParams_rear(50);
rEy1 = TireParams_rear(51);
rEy2 = TireParams_rear(52);
rHy1 = TireParams_rear(53);
rHy2 = TireParams_rear(54);
FzRL0 = TireParams_rear(55);
FzRR0 = TireParams_rear(55);
qHz1 = TireParams_rear(56);
qHz2 = TireParams_rear(57);
qHz3 = TireParams_rear(58);
qHz4 = TireParams_rear(59);
qBz1 = TireParams_rear(60);
qBz2 = TireParams_rear(61);
qBz3 = TireParams_rear(62);
qBz4 = TireParams_rear(63);
qBz5 = TireParams_rear(64);
qCz1 = TireParams_rear(65);
qDz1 = TireParams_rear(66);
qDz2 = TireParams_rear(67);
qDz3 = TireParams_rear(68);
qDz4 = TireParams_rear(69);
qEz1 = TireParams_rear(70);
qEz2 = TireParams_rear(71);
qEz3 = TireParams_rear(72);
qEz4 = TireParams_rear(73);
qEz5 = TireParams_rear(74);
qBz9 = TireParams_rear(75);
qBz10 = TireParams_rear(76);
qDz6 = TireParams_rear(77);
qDz7 = TireParams_rear(78);
qDz8 = TireParams_rear(79);
qDz9 = TireParams_rear(80);
R0 = TireParams_rear(81);
z7 = TireParams_rear(82);
ssz1 = TireParams_rear(83);
ssz2 = TireParams_rear(84);
ssz3 = TireParams_rear(85);
ssz4 = TireParams_rear(86);
qsy1 = TireParams_rear(87);
qsy2 = TireParams_rear(88);
qsy3 = TireParams_rear(89);
qsy4 = TireParams_rear(90);
Vref = TireParams_rear(91);
epsilonk = 10e-12;
%% Deviation
dFzRL = (FzRL - FzRL0)/FzRL0;
dFzRR = (FzRR - FzRR0)/FzRR0;

%% Rear Left Tire

%-------------------------------------------------------------------------%
%                      PURE LONGITUDINAL                    %
%-------------------------------------------------------------------------%
% Horizontal offset to the force/slip function of load
ShxRL   = pHx1 + pHx2.*dFzRL; 
% Longitudinal coefficient of friction in function of load
mux1RL  = (pDx1 + pDx2.*dFzRL); 
% Peak factor
DxRL    = mux1RL*FzRL; 
% Longitudinal slip ratio with offset
KxRL    = sRLx + ShxRL; 
% Shape factor
CxRL   = pCx1; 
% Curvature factor function of load
ExRL    = (pEx1 + pEx2*dFzRL + pEx3*dFzRL*dFzRL)*(1 - pEx4.*sign(KxRL)); 
% Slip stiffness Kfx/Fz function of load
KxkRL   = FzRL*(pKx1 + pKx2.*dFzRL)*exp(pKx3.*dFzRL); 
% Stiffness factor
BxRL    = KxkRL/(CxRL*DxRL + ex); 
% Vertical offset to the force/slip function of load
SVxRL   = FzRL.*(pVx1 + pVx2.*dFzRL); 
% Longitudinal Force:
Fx0RL = DxRL*sin(CxRL*atan(BxRL*KxRL - ExRL*(BxRL*KxRL - atan(BxRL*KxRL)))) + SVxRL;

%-------------------------------------------------------------------------%
%                      PURE LATERAL                    %
%-------------------------------------------------------------------------%
% Slip stiffness Kfx/Fz function of load
% Kyalf   = pKy1.*Fztlf0.*sin(pKy4.*atan(Fztlf./(pKy2+pKy5.*gammalf.^2)./Fztlf0))./(1+pKy3.*abs(gammalf));  % from book 
KyaRL = pKy1.*FzRL0.*sin(2*atan(FzRL/(pKy2*FzRL0)))*(1-pKy3*abs(gammaRL)); %Instead of sign, I put abs
% Kyglf   = (pKy6 + pKy7.*dFztlf).*Fztlf;
% Vertical offset to the force/slip function of load
SVygRL  = FzRL*(pVy3 + pVy4.*dFzRL).*gammaRL;
SVyRL   = FzRL*(pVy1 + pVy2.*dFzRL) + SVygRL; 
% Horizontal offset to the force/slip function of load
% Shlfy   = (pHy1 + pHy2.*dFztlf)+ (Kyglf.*gammalf - Svyglf)./(Kyalf +10^-6); %from book
SHyRL = (pHy1 + pHy2.*dFzRL) + pHy3.*gammaRL; %from Carmaker
% Lateral coefficient of friction in function of load
muy1RL  = (pDy1 + pDy2*dFzRL)/(1 - pDy3.*gammaRL^2);
% Peak factor
DyRL    = muy1RL*FzRL; 
% Lateral slip ratio
ayRL    = sRLy + SHyRL; 
% Shape factor
CyRL    = pCy1; 
% Curvature factor function of load
EyRL    = (pEy1 + pEy2.*dFzRL).*(1 -(pEy3+pEy4.*gammaRL).*sign(ayRL)); 
% Stiffness factor
ByRL    = KyaRL/(CyRL*DyRL + ey); 
% Lateral Force:
Fy0RL = DyRL*sin(CyRL*atan(ByRL*ayRL - EyRL*(ByRL*ayRL - atan(ByRL*ayRL)))) + SVyRL;

%-------------------------------------------------------------------------%
%                    COMBINED LONGITUDINAL                  %
%-------------------------------------------------------------------------%
BxaRL = rBx1.*cos(atan(rBx2.*sRLx));
CxaRL = rCx1;
ExaRL = rEx1 + rEx2.*dFzRL;
SHxaRL = rHx1;
aRL = sRLy + SHxaRL;
Gxa0RL = cos(CxaRL*(atan(BxaRL*SHxaRL - ExaRL*(BxaRL*SHxaRL - atan(BxaRL*SHxaRL)))));
GxaRL = (cos(CxaRL*(atan(BxaRL*aRL - ExaRL*(BxaRL*aRL - atan(BxaRL*aRL))))))/Gxa0RL;
fRLx = GxaRL*Fx0RL;

%-------------------------------------------------------------------------%
%                       COMBINED LATERAL                     %
%-------------------------------------------------------------------------%

BykRL = rBy1*cos(atan(rBy2*(sRLy-rBy3)));
CykRL = rCy1;
DVykRL = muy1RL*FzRL*(rVy1+rVy2*dFzRL + rVy3*gammaRL)*cos(atan(rVy4*sRLy));
EykRL = rEy1 + rEy2*dFzRL;
SHykRL = rHy1 + rHy2*dFzRL;
SVykRL= DVykRL*sin(rVy5*atan(rVy6*sRLx));
KsRL = sRLx + SHykRL;
Gy0kRL = cos(CykRL*atan(BykRL*SHykRL - EykRL*(BykRL*SHykRL - atan(BykRL*SHykRL))));
GykRL = cos(CykRL*atan(BykRL*KsRL - EykRL*(BykRL*KsRL - atan(BykRL*KsRL))))/Gy0kRL;
fRLy = GykRL*Fy0RL+SVykRL;

%-------------------------------------------------------------------------%
%                       PURE ALIGNING TORQUE                     %
%-------------------------------------------------------------------------%

Dr = FzRL*R0*((qDz6+qDz7*dFzRL)+(qDz8+qDz9*dFzRL)*gammaRL)-1;
SHtRL = qHz1+ qHz2*dFzRL+(qHz3+qHz4*dFzRL)*gammaRL;
at = sRLy + SHtRL;
Br = (qBz9+qBz10*ByRL*CyRL);
Dt0 = FzRL*(R0/FzRL0)*(qDz1+qDz2*dFzRL);
Dt = Dt0*(1+qDz3*gammaRL+qDz4*gammaRL^2);
Ct = qCz1;
Bt = (qBz1+qBz2*dFzRL+qBz3*dFzRL^2)*(1+qBz4*gammaRL+qBz5*abs(gammaRL));
Et = (qEz1+qEz2*dFzRL+qEz3*dFzRL^2)*(1+(qEz4+qEz5*gammaRL)*2/pi*atan(Bt*Ct*at));
Kya_primeRL = KyaRL+epsilonk;
SHfRL = SHyRL + SVyFR/Kya_primeRL;
ar = sRLy+SHfRL;
Cr = z7;
Mzr0RL = Dr*cos(Cr*atan(Br*ar))*cos(sRLy);
t0RL = Dt*cos(Ct*atan(Bt*at - Et*(Bt*at - atan(Bt*at))))*cos(sRLy);
Mz0_primeRL = -t0RL*Fy0RL;
Mz0RL = Mz0_primeRL + Mzr0RL;


%-------------------------------------------------------------------------%
%                       COMBINED ALIGNING TORQUE             %
%-------------------------------------------------------------------------%

areg = atan(sqrt(tan(ar)^2+(KxkRL/Kya_primeRL)^2*sRLx^2))*sign(ar);
ateg = atan(sqrt(tan(at)^2+(KxkRL/Kya_primeRL)^2*sRLx^2))*sign(at);
s = R0*(ssz1+ssz2*(fRLy/FzRL0)+(ssz3+ssz4*dFzRL))*gammaRL;
MzrRL = Dr*cos(Cr*atan(Br*areg))*cos(sRLy);
Fy_primeRL = fRLy - SVykRL;
t = Dt*cos(Ct*atan(Bt*ateg-Et*(Bt*ateg - atan(Bt*ateg))))*cos(sRLy);
Mz_primeRL = -t*Fy_primeRL;
mRLz = Mz_primeRL+MzrRL+s*fRLx;

%-------------------------------------------------------------------------%
%                       ROLLING RESISTANCE TORQUE             %
%-------------------------------------------------------------------------%

mRLy = -FzFR*R0*(qsy1+qsy2*(fFRx/FzFR0)+qsy3*(VFRx/Vref)+qsy4*(VFRx/Vref)^4);


%% Rear Right Tire

%-------------------------------------------------------------------------%
%                      PURE LONGITUDINAL                    %
%-------------------------------------------------------------------------%
% Horizontal offset to the force/slip function of load
ShxRR   = pHx1 + pHx2.*dFzRR; 
% Longitudinal coefficient of friction in function of load
mux1RR  = (pDx1 + pDx2.*dFzRR); 
% Peak factor
DxRR    = mux1RR*FzRR; 
% Longitudinal slip ratio with offset
KxRR    = sRRx + ShxRR; 
% Shape factor
CxRR   = pCx1; 
% Curvature factor function of load
ExRR    = (pEx1 + pEx2*dFzRR + pEx3*dFzRL*dFzRR)*(1 - pEx4.*sign(KxRR)); 
% Slip stiffness Kfx/Fz function of load
KxkRR   = FzRR*(pKx1 + pKx2.*dFzRR)*exp(pKx3.*dFzRR); 
% Stiffness factor
BxRR    = KxkRR/(CxRR*DxRR + ex); 
% Vertical offset to the force/slip function of load
SVxRR  = FzRR0*(pVx1 + pVx2.*dFzRR); 
% Longitudinal Force:
Fx0RR = DxRR*sin(CxRR*atan(BxRR*KxRR - ExRR*(BxRR*KxRR - atan(BxRR*KxRR)))) + SVxRR;

%-------------------------------------------------------------------------%
%                      PURE LATERAL                    %
%-------------------------------------------------------------------------%
% Slip stiffness Kfx/Fz function of load
% Kyalf   = pKy1.*Fztlf0.*sin(pKy4.*atan(Fztlf./(pKy2+pKy5.*gammalf.^2)./Fztlf0))./(1+pKy3.*abs(gammalf));  % from book 
KyaRR = pKy1.*FzRR0.*sin(2*atan(FzRR/(pKy2*FzRR0)))*(1-pKy3*abs(gammaRR)); %Instead of sign, I put abs
% Kyglf   = (pKy6 + pKy7.*dFztlf).*Fztlf;
% Vertical offset to the force/slip function of load
SVygRR  = FzRR*(pVy3 + pVy4.*dFzRR).*gammaRR;
SVyRR   = FzRR*(pVy1 + pVy2.*dFzRR) + SVygRR; 
% Horizontal offset to the force/slip function of load
% Shlfy   = (pHy1 + pHy2.*dFztlf)+ (Kyglf.*gammalf - Svyglf)./(Kyalf +10^-6); %from book
SHyRR = (pHy1 + pHy2.*dFzRR) + pHy3.*gammaRR; %from Carmaker
% Lateral coefficient of friction in function of load
muy1RR  = (pDy1 + pDy2*dFzRR)/(1 - pDy3.*gammaRR^2);
% Peak factor
DyRR    = muy1RR*FzRR; 
% Lateral slip ratio
ayRR    = sRRy + SHyRR; 
% Shape factor
CyRR    = pCy1; 
% Curvature factor function of load
EyRR   = (pEy1 + pEy2.*dFzRR).*(1 -(pEy3+pEy4.*gammaRR).*sign(ayRR)); 
% Stiffness factor
ByRR    = KyaRR/(CyRR*DyRR + ey); 
% Lateral Force:
Fy0RR = DyRR*sin(CyRR*atan(ByRR*ayRR - EyRR*(ByRR*ayRR - atan(ByRR*ayRR)))) + SVyRR;

%-------------------------------------------------------------------------%
%                    COMBINED LONGITUDINAL                  %
%-------------------------------------------------------------------------%
BxaRR = rBx1.*cos(atan(rBx2.*sRRx));
CxaRR = rCx1;
ExaRR = rEx1 + rEx2.*dFzRR;
SHxaRR = rHx1;
aRR = sRRy + SHxaRR;
Gxa0RR = cos(CxaRR*(atan(BxaRR*SHxaRR - ExaRR*(BxaRR*SHxaRR - atan(BxaRR*SHxaRR)))));
GxaRR = cos(CxaRR*(atan(BxaRR*aRR - ExaRR*(BxaRR*aRR - atan(BxaRR*aRR)))))/Gxa0RR;
fRRx = GxaRR*Fx0RR;

%-------------------------------------------------------------------------%
%                       COMBINED LATERAL                     %
%-------------------------------------------------------------------------%

BykRR = rBy1*cos(atan(rBy2*(sRRy-rBy3)));
CykRR = rCy1;
DVykRR = muy1RR*FzRR*(rVy1+rVy2*dFzRR + rVy3*gammaRR)*cos(atan(rVy4*sRRy));
EykRR = rEy1 + rEy2*dFzRR;
SHykRR = rHy1 + rHy2*dFzRR;
SVykRR= DVykRR*sin(rVy5*atan(rVy6*sRRx));
KsRR = sRRx + SHykRR;
Gy0kRR = cos(CykRR*atan(BykRR*SHykRR - EykRR*(BykRR*SHykRR - atan(BykRR*SHykRR))));
GykRR = (cos(CykRR*atan(BykRR*KsRR - EykRR*(BykRR*KsRR - atan(BykRR*KsRR)))))/Gy0kRR;
fRRy = GykRR*Fy0RR+SVykRR;

%-------------------------------------------------------------------------%
%                       PURE ALIGNING TORQUE                     %
%-------------------------------------------------------------------------%

Dr = FzRR*R0*((qDz6+qDz7*dFzRR)+(qDz8+qDz9*dFzRR)*gammaRR)-1;
SHtRR = qHz1+ qHz2*dFzRR+(qHz3+qHz4*dFzRR)*gammaRR;
at = sRRy + SHtRR;
Br = (qBz9+qBz10*ByRR*CyRR);
Dt0 = FzRR*(R0/FzRR0)*(qDz1+qDz2*dFzRR);
Dt = Dt0*(1+qDz3*gammaRR+qDz4*gammaRR^2);
Ct = qCz1;
Bt = (qBz1+qBz2*dFzRR+qBz3*dFzRR^2)*(1+qBz4*gammaRR+qBz5*abs(gammaRR));
Et = (qEz1+qEz2*dFzRR+qEz3*dFzRR^2)*(1+(qEz4+qEz5*gammaRR)*2/pi*atan(Bt*Ct*at));
Kya_primeRR = KyaRR+epsilonk;
SHfRR = SHyRR + SVyFR/Kya_primeRR;
ar = sRRy+SHfRR;
Cr = z7;
Mzr0RR = Dr*cos(Cr*atan(Br*ar))*cos(sRRy);
t0RR = Dt*cos(Ct*atan(Bt*at - Et*(Bt*at - atan(Bt*at))))*cos(sRRy);
Mz0_primeRR = -t0RR*Fy0RR;
Mz0RR = Mz0_primeRR + Mzr0RR;


%-------------------------------------------------------------------------%
%                       COMBINED ALIGNING TORQUE             %
%-------------------------------------------------------------------------%

areg = atan(sqrt(tan(ar)^2+(KxkRR/Kya_primeRR)^2*sRRx^2))*sign(ar);
ateg = atan(sqrt(tan(at)^2+(KxkRR/Kya_primeRR)^2*sRRx^2))*sign(at);
s = R0*(ssz1+ssz2*(fRRy/FzRR0)+(ssz3+ssz4*dFzRR))*gammaRR;
MzrRR = Dr*cos(Cr*atan(Br*areg))*cos(sRRy);
Fy_primeRR = fRRy - SVykRR;
t = Dt*cos(Ct*atan(Bt*ateg-Et*(Bt*ateg - atan(Bt*ateg))))*cos(sRRy);
Mz_primeRR = -t*Fy_primeRR;
mRRz = Mz_primeRR+MzrRR+s*fRRx;

%-------------------------------------------------------------------------%
%                       ROLLING RESISTANCE TORQUE             %
%-------------------------------------------------------------------------%

mRRy = -FzFR*R0*(qsy1+qsy2*(fFRx/FzFR0)+qsy3*(VFRx/Vref)+qsy4*(VFRx/Vref)^4);

%% Wheel Dynamics
domegaFL = (TFL - fFLx*rF)/(JwF);
domegaFR = (TFR - fFRx*rF)/(JwF);
domegaRL = (TRL - fRLx*rR)/(JwR);
domegaRR = (TRR - fRRx*rR)/(JwR);

omega_dot = [domegaFL, domegaFR, domegaRL, domegaRR];

end

== matlab function VDSE_2019b1/ROAD PROFILE/GENERATION OF ROAD PROFILE ==
  data: sim_time input; yFL_road output; bump_height input; bump_length input; lF input; lR input; bump_time input; Vx input; yFR_road output; yRL_road output; yRR_road output
function [yFL_road,yFR_road,yRL_road,yRR_road]  = Road(sim_time, bump_height,bump_length,lF,lR,bump_time,Vx)
lag= (lF+lR)/Vx;
ww=2*pi*Vx/bump_length;
if sim_time>=bump_time & sim_time<(bump_length/Vx)+bump_time
    yFL_road=bump_height/2*(1-cos(ww*(sim_time-bump_time)));
    yFR_road=bump_height/2*(1-cos(ww*(sim_time-bump_time)));
else
    yFL_road=0;
    yFR_road=0;
end
lag=(lF+lR)/Vx;
if sim_time>=lag+bump_time & sim_time<(lag+bump_length/Vx)+bump_time
    yRL_road=bump_height/2*(1-cos(ww*(sim_time-lag-bump_time)));
    yRR_road=bump_height/2*(1-cos(ww*(sim_time-lag-bump_time)));
else
    yRL_road=0;
    yRR_road=0;
end
end
